simulink model "test_motors"  (R2023a)
settings: Solver=FixedStepAuto  StartTime=0.0  StopTime=inf  FixedStep=0.01  RelTol=1e-3  EnableMultiTasking=on
undefined symbols (not defined in the file): AUX, dev, Main, pwm_output0, pwm_output1
libraries: px4lib x2, px4uORBlib x1, simulink x1
settings Model: SimulationMode=external  ExtModeTrigDuration=10  Creator=ArriGE66  LastModifiedBy=ArriGE66
settings SolverCC: PositivePriorityOrder=on
settings OptimizationCC: EnhancedBackFolding=on  PassReuseOutputArgsAs=Individual arguments  ZeroExternalMemoryAtStartup=off  ZeroInternalMemoryAtStartup=off  MaxStackSize=64  OptimizeBlockOrder=speed  DifferentSizesBufferReuse=on  OptimizationCustomize=off  EfficientTunableParamExpr=on
settings DebuggingCC: ParameterTunabilityLossMsg=error
settings HardwareCC: ProdBitPerPointer=32  ProdBitPerSizeT=32  ProdBitPerPtrDiffT=32  ProdLargestAtomicInteger=Long  ProdLargestAtomicFloat=Double  ProdWordSize=32  ProdLongLongMode=on  ProdHWDeviceType=ARM Compatible->ARM Cortex
settings SFSimCC: MATLABDynamicMemAlloc=off  SimTargetLang=C++
settings RTWCC: Description=Embedded Coder  SystemTargetFile=ert.tlc  HardwareBoard=PX4 Cube Orange  TemplateMakefile=ert_default_tmf  Toolchain=GNU Tools for PX4 Autopilots  TargetLang=C++
settings CodeAppCC: ForceParamTrailComments=on  IgnoreCustomStorageClasses=off  OperatorAnnotations=on  SimulinkDataObjDesc=on  SFDataObjDesc=on  InsertBlockDesc=on
settings ERTTargetCC: ExtMode=on  ExtModeTransport=3  ExtModeStaticAlloc=on  ExtModeStaticAllocSize=1024  ExtModeMexFile=ext_xcp  ExtModeMexArgs=1 COM10 3000000  ExtModeIntrfLevel=Level2 - Open

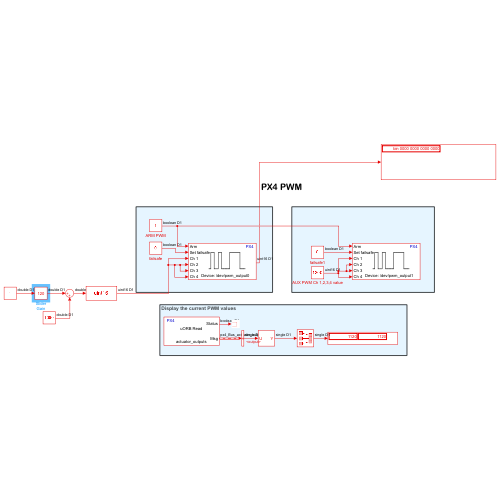
[thumbnail: Simulink's stored preview of the top-level diagram]
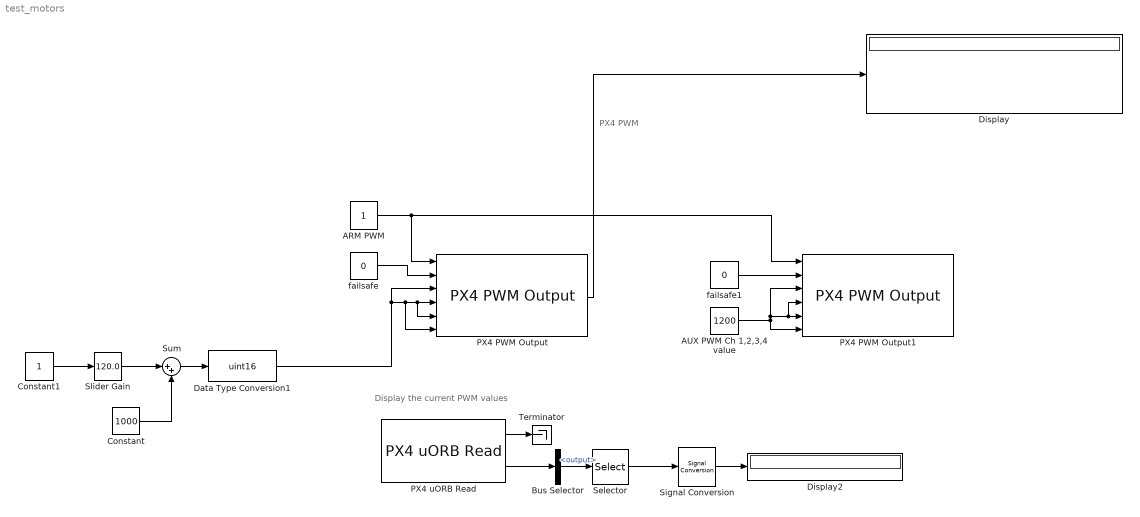
== system test_motors ==
  note: PX4 PWM
  note: Display the current PWM values
  ARM PWM : Constant  OutDataTypeStr=boolean  SampleTime=0.01
  AUX PWM Ch 1,2,3,4 value : Constant  Value=1200  OutDataTypeStr=uint16  SampleTime=0.01
  Bus Selector : BusSelector  OutputSignals=output
  Constant : Constant  Value=1000  SampleTime=0.01
  Constant1 : Constant  SampleTime=0.01
  Data Type Conversion1 : DataTypeConversion  OutDataTypeStr=uint16  SaturateOnIntegerOverflow=off  RndMeth=Floor
  Display : Display
      settings: Format=binary (Stored Integer)
  Display2 : Display
  PX4 PWM Output : px4lib/PX4 PWM Output  pwmDevice=Main (/dev/pwm_output0)  pwmChannel1_=on  pwmChannel2_=on  pwmChannel3_=on  pwmChannel4_=on  pwmChannel5_=off  pwmChannel6_=off  pwmChannel7_=off  pwmChannel8_=off  forceTerminateFailsafe=off  outputErrorStatus=on
  PX4 PWM Output1 : px4lib/PX4 PWM Output  pwmDevice=AUX (/dev/pwm_output1)  pwmChannel1_=on  pwmChannel2_=on  pwmChannel3_=on  pwmChannel4_=on  pwmChannel5_=off  pwmChannel6_=off  pwmChannel7_=off  pwmChannel8_=off  forceTerminateFailsafe=off  outputErrorStatus=off
  PX4 uORB Read : px4uORBlib/PX4 uORB Read  uORBTopic=actuator_outputs  selectInstance=actuator_outputs  SampleTime=0.01  BlockingMode=off  BlockTimeout=1e-3
  Selector : Selector  InputPortWidth=16  IndexOptions=Index vector (dialog)  Indices=[1 2]  OutputSizes=1
  Signal Conversion : SignalConversion  OverrideOpt=off
  Slider Gain : simulink/Math Operations/Slider Gain  gain=120.0  low=0  high=1000
  Sum : Sum  Inputs=|++
  Terminator : Terminator
  failsafe : Constant  Value=0  OutDataTypeStr=boolean  SampleTime=0.01
  failsafe1 : Constant  Value=0  OutDataTypeStr=boolean  SampleTime=0.01
  wires:
  ARM PWM/1 -> PX4 PWM Output1/1, PX4 PWM Output/1
  Data Type Conversion1/1 -> PX4 PWM Output/6, PX4 PWM Output/5, PX4 PWM Output/4, PX4 PWM Output/3
  Bus Selector/1 -> Selector/1  "<output>"
  PX4 uORB Read/1 -> Terminator/1
  failsafe/1 -> PX4 PWM Output/2
  Selector/1 -> Signal Conversion/1
  AUX PWM Ch 1,2,3,4 value/1 -> PX4 PWM Output1/3, PX4 PWM Output1/5, PX4 PWM Output1/4, PX4 PWM Output1/6
  PX4 uORB Read/2 -> Bus Selector/1
  failsafe1/1 -> PX4 PWM Output1/2
  Signal Conversion/1 -> Display2/1
  Slider Gain/1 -> Sum/1
  Constant/1 -> Sum/2
  Constant1/1 -> Slider Gain/1
  Sum/1 -> Data Type Conversion1/1
  PX4 PWM Output/1 -> Display/1
